simulink model "chap5_3sim"  (Simulink 7.7)
settings: Solver=ode45  StartTime=0.0  StopTime=20  FixedStep=0.001  RelTol=1e-3
settings Model: Creator=hp  LastModifiedBy=ljk  ExtModeTrigMode=oneshot  ExtModeArmWhenConnect=off
settings DataIOCC: LimitDataPoints=off  SignalLoggingName=sigsOut
settings OptimizationCC: BooleanDataType=off  InitFltsAndDblsToZero=on
settings DebuggingCC: SaveWithParameterizedLinksMsg=none  SignalResolutionControl=TryResolveAllWithWarning  SolverPrmCheckMsg=none  MultiTaskDSMMsg=warning  MultiTaskCondExecSysMsg=none  StrictBusMsg=None
settings HardwareCC: TargetUnknown=on
settings RTWCC: IncludeERTFirstTime=on
settings GRTTargetCC: TargetFcnLib=ansi_tfl_tmw.mat

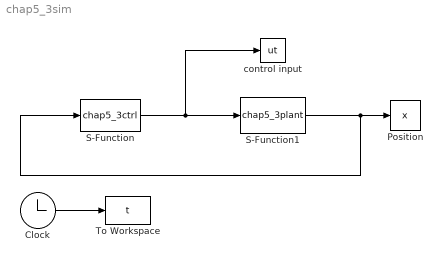
== system chap5_3sim ==
  Clock : Clock
      settings: Decimation=10
  Position : ToWorkspace  VariableName=x  SampleTime=-1  SaveFormat=Array
  S-Function : S-Function  FunctionName=chap5_3ctrl  EnableBusSupport=off
  S-Function1 : S-Function  FunctionName=chap5_3plant  EnableBusSupport=off
  To Workspace : ToWorkspace  VariableName=t  SampleTime=-1  SaveFormat=Array
  control input : ToWorkspace  VariableName=ut  SampleTime=-1  SaveFormat=Array
  wires:
  S-Function/1 -> S-Function1/1, control input/1
  S-Function1/1 -> S-Function/1, Position/1
  Clock/1 -> To Workspace/1
